simulink model "maszyna_atwooda"  (R2024b)
settings: Solver=ode45  StartTime=0.0  StopTime=50  MaxStep=2^-5  RelTol=1e-3
libraries: simulink x2
settings Model: Creator=kg53848  LastModifiedBy=kg53848

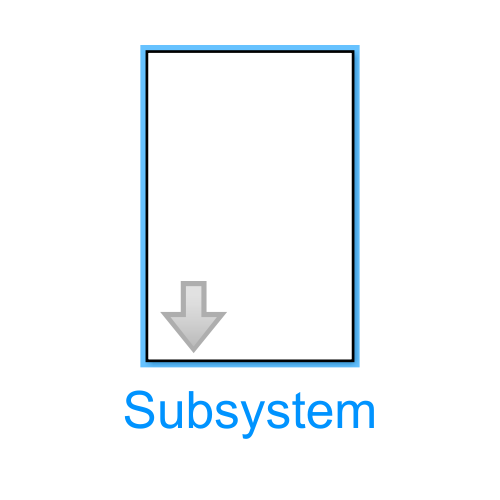
[thumbnail: Simulink's stored preview of the top-level diagram]
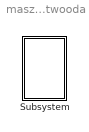
== system maszyna_atwooda ==
  Subsystem : Subsystem  mask{g=9.81, m1=2.2, m2=2, M=3, R=0.002, r0=2, theta0=45}
      mask prompts: g "przysp"; m1 "masa wahadla"; m2 "masa ciezarka"; M "masa bloczkow"; R "promien bloczkow"; r0 "poczatkowa dlugosc linki wahadla"; theta0 "poczatkowy kat"

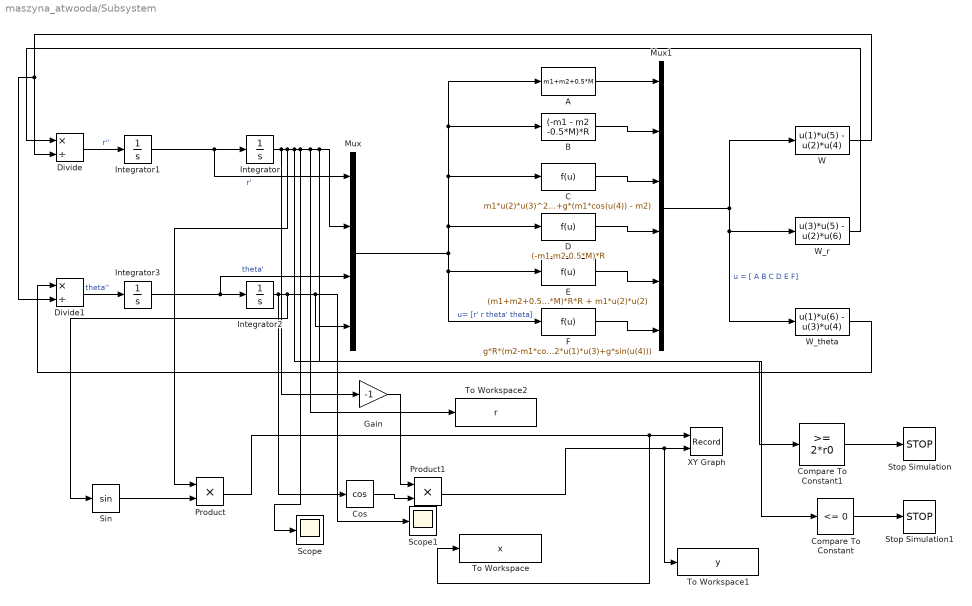
== system maszyna_atwooda/Subsystem ==
  A : Fcn  Expr=m1+m2+0.5*M
  B : Fcn  Expr=(-m1 - m2 -0.5*M)*R
  C : Fcn  Expr=m1*u(2)*u(3)^2+g*(m1*cos(u(4)) - m2)
  Compare To Constant : simulink/Logic and Bit Operations/Compare To Constant  relop=<=  const=0  OutDataTypeStr=boolean
  Compare To Constant1 : simulink/Logic and Bit Operations/Compare To Constant  relop=>=  const=2*r0  OutDataTypeStr=boolean
  Cos : Trigonometry  Operator=cos
  D : Fcn  Expr=(-m1-m2-0.5*M)*R
  Divide : Product  Inputs=*/
  Divide1 : Product  Inputs=*/
  E : Fcn  Expr=(m1+m2+0.5*M)*R*R + m1*u(2)*u(2)
  F : Fcn  Expr=g*R*(m2-m1*cos(u(4)))-m1*u(2)*(2*u(1)*u(3)+g*sin(u(4)))
  Gain : Gain  Gain=-1
  Integrator : Integrator  InitialCondition=r0
  Integrator1 : Integrator
  Integrator2 : Integrator  InitialCondition=theta0*pi/180
  Integrator3 : Integrator
  Mux : Mux
  Mux1 : Mux  Inputs=6
  Product : Product
  Product1 : Product
  Scope : Scope
  Scope1 : Scope
  Sin : Trigonometry
  Stop Simulation : Stop
  Stop Simulation1 : Stop
  To Workspace : ToWorkspace  VariableName=x  SampleTime=-1
  To Workspace1 : ToWorkspace  VariableName=y  SampleTime=-1
  To Workspace2 : ToWorkspace  VariableName=r  SampleTime=-1
  W : Fcn  Expr=u(1)*u(5) - u(2)*u(4)
  W_r : Fcn  Expr=u(3)*u(5) - u(2)*u(6)
  W_theta : Fcn  Expr=u(1)*u(6) - u(3)*u(4)
  XY Graph : Record  FileSettingsInternal="{\"entries\":[{\"content\":{\"excelSettings\":{\"content\":{},\"type\":\"Streamout.ExcelSettings\"}},\"type\":\"Streamout.FileSettingStorage\",\"uuid\":\"\"}],\"packageUris\":[\"http:\\/\\/schema.mathworks.com\\/mf0\\/streamout_blocks\\/R2020a\"],\"version\":\"1.0\"}"  Layout=[1 1]  SignalsInternal="{\"entries\":[{\"content\":{\"signals\":[{\"content\":{\"blockPath\":[],\"dimensions\":[1],\"domain\":\"\",\"lineColor\":\"#a2142f\",\"plots\":[ 1 ],\"port\":1,\"sid\":[\"\"],\"signalID\":1,\"signalName\":\"Product\"},\"type\":\"RecordBlkView.Signal\",\"uuid\":\"\"},{\"content\":{\"blockPath\":[],\"dimensions\":[1],\"domain\":\"\",\"lineColor\":\"#139fff\",\"plots\":[ 1 ],\"port\":2,\"sid\":[\"\"],\"signalID\":2,\"signalName\":\"Product1\"},\"type\":\"RecordBlkView.Signal\",\"uuid\":\"\"}]},\"type\":\"RecordBlkView.InputSignals\",\"uuid\":\"\"}],\"packageUris\":[\"http:\\/\\/schema.mathworks.com\\/mf0\\/streamout_blocks\\/R2020a\"],\"version\":\"1.0\"}"  VisualizationBindings="{\"xyplotplugin\":{\"info\":[{\"series\":[{\"bindingParametersList\":[{\"parameter\":\"X-Axis\",\"signalID\":1,\"signalName\":\"Product\"},{\"parameter\":\"Y-Axis\",\"signalID\":2,\"signalName\":\"Product1\"}],\"seriesID\":0}],\"subplotID\":1}]}}"  CompatibilityTag=XY
  wires:
  Mux1/1 -> W_theta/1, W_r/1, W/1  "u = [ A B C D E F]"
  Mux/1 -> E/1, F/1, B/1, A/1, C/1, D/1  "u= [r' r theta' theta]"
  Integrator1/1 -> Mux/1, Integrator/1  "r'"
  Integrator/1 -> Gain/1, Product/1, Compare To Constant/1, Scope/1, To Workspace2/1, Compare To Constant1/1, Mux/2
  Product/1 -> To Workspace/1, XY Graph/1
  Integrator3/1 -> Mux/3, Integrator2/1  "theta'"
  Divide/1 -> Integrator1/1  "r''"
  E/1 -> Mux1/5
  Integrator2/1 -> Cos/1, Sin/1, Mux/4, Scope1/1
  Divide1/1 -> Integrator3/1  "theta''"
  W/1 -> Divide1/2, Divide/2
  Sin/1 -> Product/2
  A/1 -> Mux1/1
  D/1 -> Mux1/4
  W_theta/1 -> Divide1/1
  F/1 -> Mux1/6
  C/1 -> Mux1/3
  B/1 -> Mux1/2
  Product1/1 -> To Workspace1/1, XY Graph/2
  W_r/1 -> Divide/1
  Gain/1 -> Product1/1
  Cos/1 -> Product1/2
  Compare To Constant1/1 -> Stop Simulation/1
  Compare To Constant/1 -> Stop Simulation1/1
